simulink model "symulink2"  (Simulink 7.2)
settings: Solver=ode45  StartTime=0.0  StopTime=10.0  RelTol=1e-3
values from neighbouring files (symbols this model uses):
  Beq = 2.5821e-4    (= 0.00025821)    [GlobalParam.m]
  Jeq = 7.7463e-4    (= 0.00077463)    [GlobalParam.m]
settings Model: Creator=ALan  LastModifiedBy=ALan

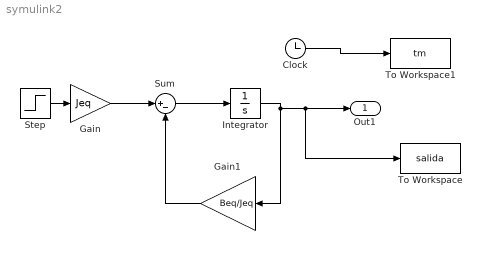
== system symulink2 ==
  Clock : Clock
      settings: Decimation=10
  Gain : Gain  Gain=Jeq  ParameterDataType=sfix(16)  ParameterScaling=2^0  OutDataType=sfix(16)  OutScaling=2^0
  Gain1 : Gain  Orientation=left  Gain=Beq/Jeq  ParameterDataType=sfix(16)  ParameterScaling=2^0  OutDataType=sfix(16)  OutScaling=2^0
  Integrator : Integrator
  Step : Step  SampleTime=0
  Sum : Sum  Inputs=|+-  OutDataType=sfix(16)  OutScaling=2^0
  To Workspace : ToWorkspace  VariableName=salida  SampleTime=-1  SaveFormat=Array
  To Workspace1 : ToWorkspace  VariableName=tm  SampleTime=-1  SaveFormat=Array
  Out1 : Outport  OutDataType=sfix(16)  OutScaling=2^0
  wires:
  Sum/1 -> Integrator/1
  Integrator/1 -> Gain1/1, Out1/1, To Workspace/1
  Gain1/1 -> Sum/2
  Gain/1 -> Sum/1
  Clock/1 -> To Workspace1/1
  Step/1 -> Gain/1
